simulink model "leg_ctrl"  (R2023a)
settings: Solver=VariableStepAuto  StartTime=0.0  StopTime=12  RelTol=1e-3
values from neighbouring files (symbols this model uses):
  AT = double(subs(A,E,F(i,1:11)))    [leg_ctrl.m]
  BT = double(subs(B,E, F(i, 1:11)))    [leg_ctrl.m]
  K_L0 = double(subs(K_L0,L0,0.280684+0.111146))    [leg_ctrl.m]
settings Model: Creator=Lenovo  LastModifiedBy=Lenovo

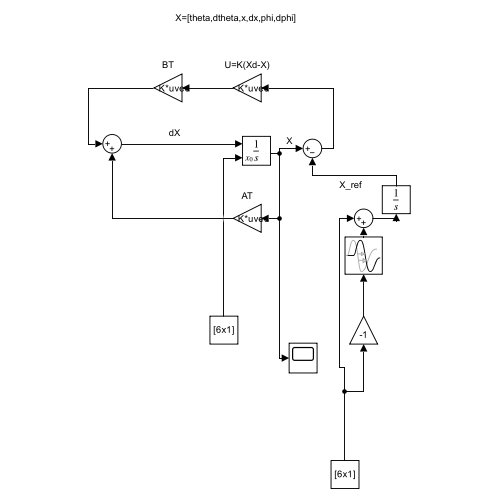
[thumbnail: Simulink's stored preview of the top-level diagram]
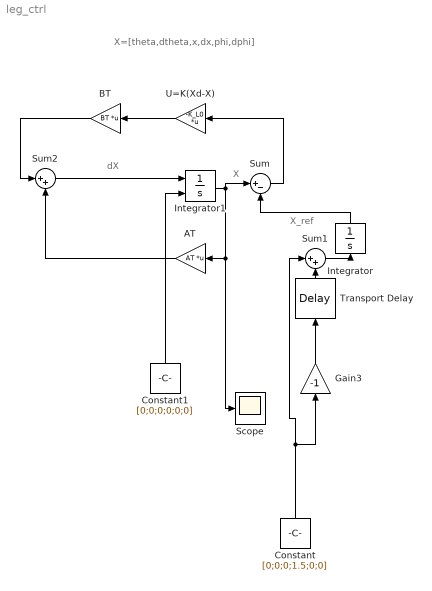
== system leg_ctrl ==
  note: X=[theta,dtheta,x,dx,phi,dphi]
  note: X_ref
  note: X
  note: dX
  AT : Gain  Gain=AT  Multiplication=Matrix(K*u) (u vector)
  BT : Gain  Gain=BT  Multiplication=Matrix(K*u) (u vector)
  Constant : Constant  Value=[0;0;0;1.5;0;0]  VectorParams1D=off  SampleTime=3
  Constant1 : Constant  Value=[0;0;0;0;0;0]  VectorParams1D=off
  Gain3 : Gain  Gain=-1
  Integrator : Integrator
  Integrator1 : Integrator  InitialConditionSource=external  InitialCondition=[0;0;0;0;0;0]
  Scope : Scope
  Sum : Sum  Inputs=|+-
  Sum1 : Sum  Inputs=|++
  Sum2 : Sum  Inputs=|++
  Transport Delay : TransportDelay  DelayTime=6
  U=K(Xd-X) : Gain  Gain=-K_L0  Multiplication=Matrix(K*u) (u vector)
  wires:
  U=K(Xd-X)/1 -> BT/1
  Integrator1/1 -> Scope/1, AT/1, Sum/1
  Constant/1 -> Sum1/1, Gain3/1
  BT/1 -> Sum2/1
  AT/1 -> Sum2/2
  Constant1/1 -> Integrator1/2
  Transport Delay/1 -> Sum1/2
  Gain3/1 -> Transport Delay/1
  Sum/1 -> U=K(Xd-X)/1
  Sum2/1 -> Integrator1/1
  Sum1/1 -> Integrator/1
  Integrator/1 -> Sum/2
